simulink model "PruebaN9_sinRap"  (R2024b)
settings: Solver=ode45  StartTime=0.0  StopTime=10  RelTol=1e-3
values from neighbouring files (symbols this model uses):
  T = 10e-3    (= 0.01)    [Proceso.m]    (also in regdiagSISOsep.m = Reg.Ts; regdiagsep.m = Reg.Ts; regsep.m = Reg.Ts)
undefined symbols (not defined in the file or in its folder): N, RegDiag_Len2_ext, RegDiag_Len3_ext, RegDiag_Len4_ext, RegDiag_Len5_ext, RegDiag_Len6_ext, RegDiag_Len7_ext, RegDiag_Len8_ext, RegDiag_Len9_ext
libraries: cstblocks x12
settings Model: Creator=Guillem  LastModifiedBy=jroigro
settings SolverCC: AlgebraicLoopSolver=TrustRegion
settings DataIOCC: LimitDataPoints=on  SaveFormat=Array  SignalLoggingSaveFormat=ModelDataLogs  ReturnWorkspaceOutputs=off
settings OptimizationCC: BlockReduction=off  BooleanDataType=off  LifeSpan=inf
settings DebuggingCC: SaveWithParameterizedLinksMsg=none  UnderspecifiedInitializationDetection=Classic  MergeDetectMultiDrivingBlocksExec=none  SignalResolutionControl=TryResolveAllWithWarning  MultiTaskDSMMsg=warning  MultiTaskCondExecSysMsg=none  UnconnectedInputMsg=warning  UnconnectedOutputMsg=warning  UnconnectedLineMsg=warning  SFUnexpectedBacktrackingDiag=warning  SFNoUnconditionalDefaultTransitionDiag=warning  SFExecutionAtInitializationDiag=none  ArithmeticOperatorsInVariantConditions=warning
settings HardwareCC: ProdBitPerPointer=32  ProdBitPerSizeT=32  ProdBitPerPtrDiffT=32  ProdLargestAtomicFloat=None  ProdIntDivRoundTo=Undefined  ProdEndianess=Unspecified  ProdWordSize=32  ProdHWDeviceType=32-bit Generic  TargetUnknown=on
settings ModelReferenceCC: PropagateSignalLabelsOutOfModel=off
settings SFSimCC: SimUseLocalCustomCode=off  CustomCodeUndefinedFunction=UseInterfaceOnly
settings RTWCC: RTWUseLocalCustomCode=off  GPUComputeCapability=3.5
settings CodeAppCC: StateflowObjectComments=on
settings GRTTargetCC: TargetLangStandard=C89/C90 (ANSI)
settings ConfigComp: CovMetricSettings=dw  CovSaveCumulativeToWorkspaceVar=on  CovSaveSingleToWorkspaceVar=on  CovExternalEMLEnable=off

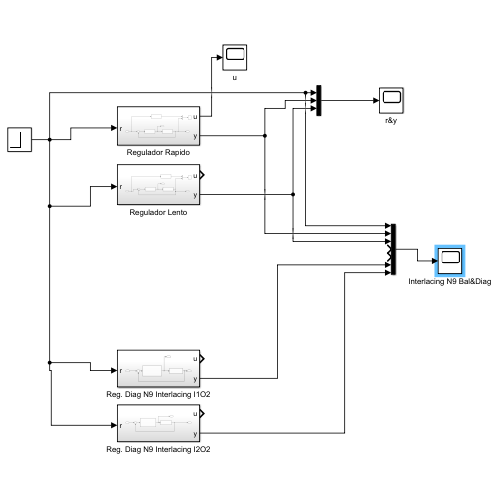
[thumbnail: Simulink's stored preview of the top-level diagram]
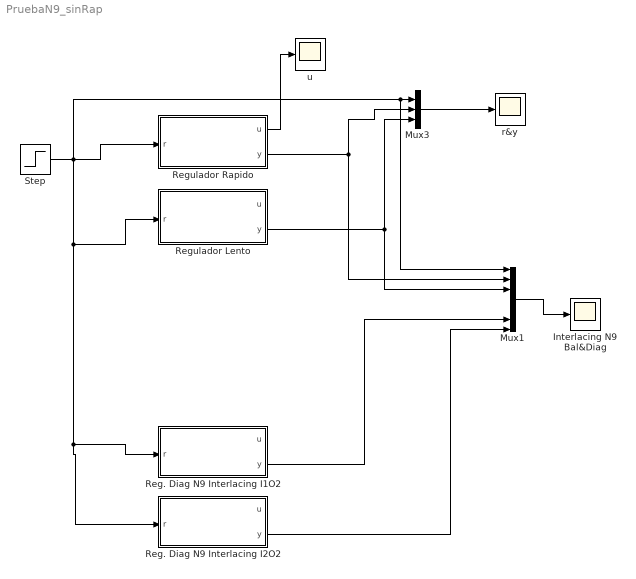
== system PruebaN9_sinRap ==
  Interlacing N9 Bal&Diag : Scope
  Mux1 : Mux  Inputs=7
  Mux3 : Mux  Inputs=3
  Reg. Diag N9 Interlacing I1O2 : Subsystem
  Reg. Diag N9 Interlacing I2O2 : Subsystem
  Regulador Lento : Subsystem
  Regulador Rapido : Subsystem
  Step : Step  Time=10  Before=1  After=2  SampleTime=0
  r&y : Scope
  u : Scope
  wires:
  Mux3/1 -> r&y/1
  Regulador Rapido/2(y) -> Mux1/2, Mux3/2
  Regulador Rapido/1(u) -> u/1
  Mux1/1 -> Interlacing N9 Bal&Diag/1
  Regulador Lento/2(y) -> Mux1/3, Mux3/3
  Step/1 -> Reg. Diag N9 Interlacing I1O2/1(r), Reg. Diag N9 Interlacing I2O2/1(r), Regulador Lento/1(r), Mux1/1, Mux3/1, Regulador Rapido/1(r)
  Reg. Diag N9 Interlacing I2O2/2(y) -> Mux1/7
  Reg. Diag N9 Interlacing I1O2/2(y) -> Mux1/6

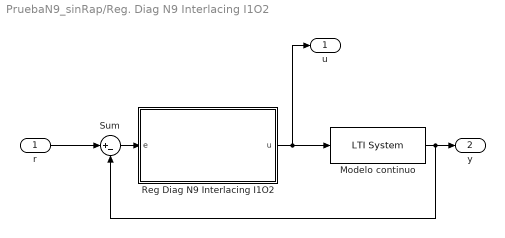
== system PruebaN9_sinRap/Reg. Diag N9 Interlacing I1O2 ==
  r : Inport
  Modelo continuo : cstblocks/LTI System  sys=Planta  IC=[]  PadeOrder=0
  Reg Diag N9 Interlacing I1O2 : Subsystem
  Sum : Sum  Inputs=|+-
  u : Outport
  y : Outport  Port=2
  wires:
  Reg Diag N9 Interlacing I1O2/1(u) -> Modelo continuo/1, u/1
  r/1 -> Sum/1
  Sum/1 -> Reg Diag N9 Interlacing I1O2/1(e)
  Modelo continuo/1 -> Sum/2, y/1

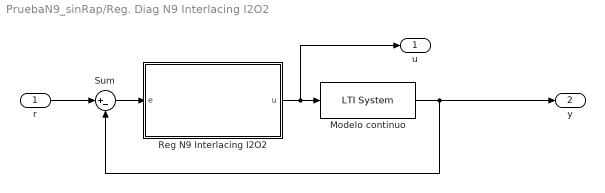
== system PruebaN9_sinRap/Reg. Diag N9 Interlacing I2O2 ==
  r : Inport
  Modelo continuo : cstblocks/LTI System  sys=Planta  IC=[]  PadeOrder=0
  Reg N9 Interlacing I2O2 : Subsystem
  Sum : Sum  Inputs=|+-
  u : Outport
  y : Outport  Port=2
  wires:
  Modelo continuo/1 -> Sum/2, y/1
  Reg N9 Interlacing I2O2/1(u) -> Modelo continuo/1, u/1
  r/1 -> Sum/1
  Sum/1 -> Reg N9 Interlacing I2O2/1(e)

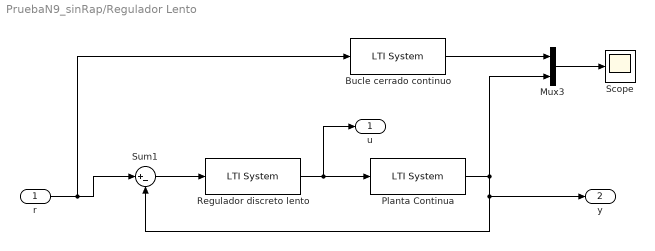
== system PruebaN9_sinRap/Regulador Lento ==
  r : Inport
  Bucle cerrado continuo : cstblocks/LTI System  sys=BC2  IC=[]  PadeOrder=0
  Mux3 : Mux  Inputs=2
  Planta Continua : cstblocks/LTI System  sys=Planta  IC=[]  PadeOrder=0
  Regulador discreto lento : cstblocks/LTI System  sys=GrN9  IC=[]  PadeOrder=0
  Scope : Scope
  Sum1 : Sum  Inputs=|+-
  u : Outport
  y : Outport  Port=2
  wires:
  r/1 -> Bucle cerrado continuo/1, Sum1/1
  Regulador discreto lento/1 -> u/1, Planta Continua/1
  Sum1/1 -> Regulador discreto lento/1
  Planta Continua/1 -> Sum1/2, y/1, Mux3/2
  Mux3/1 -> Scope/1
  Bucle cerrado continuo/1 -> Mux3/1

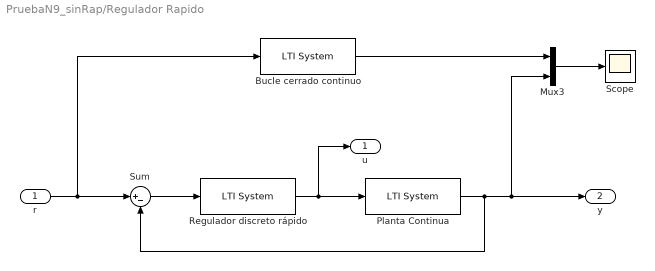
== system PruebaN9_sinRap/Regulador Rapido ==
  r : Inport
  Bucle cerrado continuo : cstblocks/LTI System  sys=BC1  IC=[]  PadeOrder=0
  Mux3 : Mux  Inputs=2
  Planta Continua : cstblocks/LTI System  sys=Planta  IC=[]  PadeOrder=0
  Regulador discreto rápido : cstblocks/LTI System  sys=Gr  IC=[]  PadeOrder=0
  Scope : Scope
  Sum : Sum  Inputs=|+-
  u : Outport
  y : Outport  Port=2
  wires:
  Regulador discreto rápido/1 -> u/1, Planta Continua/1
  Bucle cerrado continuo/1 -> Mux3/1
  Mux3/1 -> Scope/1
  Sum/1 -> Regulador discreto rápido/1
  Planta Continua/1 -> Mux3/2, y/1, Sum/2
  r/1 -> Sum/1, Bucle cerrado continuo/1

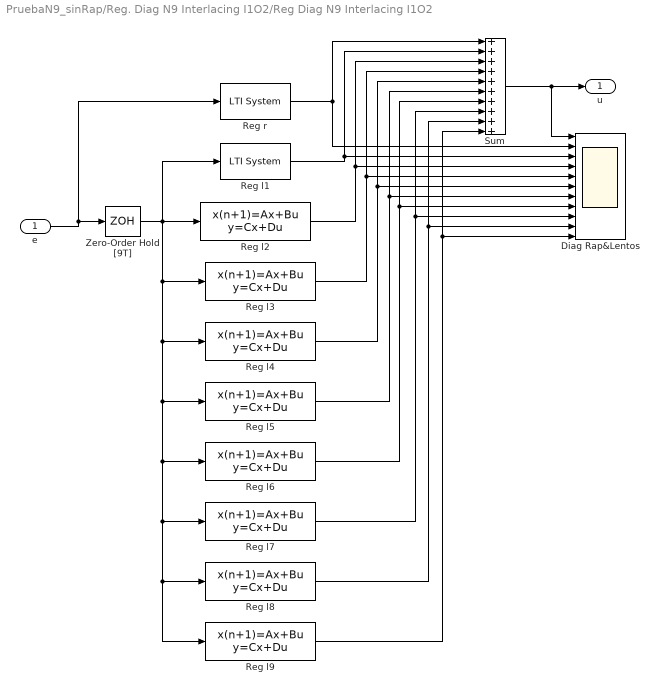
== system PruebaN9_sinRap/Reg. Diag N9 Interlacing I1O2/Reg Diag N9 Interlacing I1O2 ==
  e : Inport
  Diag Rap&Lentos : Scope  NumInputPorts=11
  Reg l1 : cstblocks/LTI System  sys=RegDiag_Len1_ext  IC=[]  PadeOrder=0
  Reg l2 : DiscreteStateSpace  A=RegDiag_Len2_ext.A  B=RegDiag_Len2_ext.B  C=RegDiag_Len2_ext.C  D=RegDiag_Len2_ext.D  SampleTime=[N*T,T]
  Reg l3 : DiscreteStateSpace  A=RegDiag_Len3_ext.A  B=RegDiag_Len3_ext.B  C=RegDiag_Len3_ext.C  D=RegDiag_Len3_ext.D  SampleTime=[N*T,2*T]
  Reg l4 : DiscreteStateSpace  A=RegDiag_Len4_ext.A  B=RegDiag_Len4_ext.B  C=RegDiag_Len4_ext.C  D=RegDiag_Len4_ext.D  SampleTime=[N*T,3*T]
  Reg l5 : DiscreteStateSpace  A=RegDiag_Len5_ext.A  B=RegDiag_Len5_ext.B  C=RegDiag_Len5_ext.C  D=RegDiag_Len5_ext.D  SampleTime=[N*T,4*T]
  Reg l6 : DiscreteStateSpace  A=RegDiag_Len6_ext.A  B=RegDiag_Len6_ext.B  C=RegDiag_Len6_ext.C  D=RegDiag_Len6_ext.D  SampleTime=[N*T,5*T]
  Reg l7 : DiscreteStateSpace  A=RegDiag_Len7_ext.A  B=RegDiag_Len7_ext.B  C=RegDiag_Len7_ext.C  D=RegDiag_Len7_ext.D  SampleTime=[N*T,6*T]
  Reg l8 : DiscreteStateSpace  A=RegDiag_Len8_ext.A  B=RegDiag_Len8_ext.B  C=RegDiag_Len8_ext.C  D=RegDiag_Len8_ext.D  SampleTime=[N*T,7*T]
  Reg l9 : DiscreteStateSpace  A=RegDiag_Len9_ext.A  B=RegDiag_Len9_ext.B  C=RegDiag_Len9_ext.C  D=RegDiag_Len9_ext.D  SampleTime=[N*T,8*T]
  Reg r : cstblocks/LTI System  sys=RegDiag_Rap  IC=[]  PadeOrder=0
  Sum : Sum  Inputs=++++++++++
  Zero-Order Hold [9T] : ZeroOrderHold  SampleTime=[N*T]
  u : Outport
  wires:
  Sum/1 -> u/1, Diag Rap&Lentos/1
  Reg l1/1 -> Sum/2, Diag Rap&Lentos/3
  Reg r/1 -> Diag Rap&Lentos/2, Sum/1
  e/1 -> Reg r/1, Zero-Order Hold [9T]/1
  Zero-Order Hold [9T]/1 -> Reg l9/1, Reg l8/1, Reg l7/1, Reg l6/1, Reg l5/1, Reg l4/1, Reg l3/1, Reg l1/1, Reg l2/1
  Reg l2/1 -> Sum/3, Diag Rap&Lentos/4
  Reg l3/1 -> Diag Rap&Lentos/5, Sum/4
  Reg l4/1 -> Sum/5, Diag Rap&Lentos/6
  Reg l5/1 -> Sum/6, Diag Rap&Lentos/7
  Reg l6/1 -> Sum/7, Diag Rap&Lentos/8
  Reg l7/1 -> Sum/8, Diag Rap&Lentos/9
  Reg l8/1 -> Diag Rap&Lentos/10, Sum/9
  Reg l9/1 -> Diag Rap&Lentos/11, Sum/10

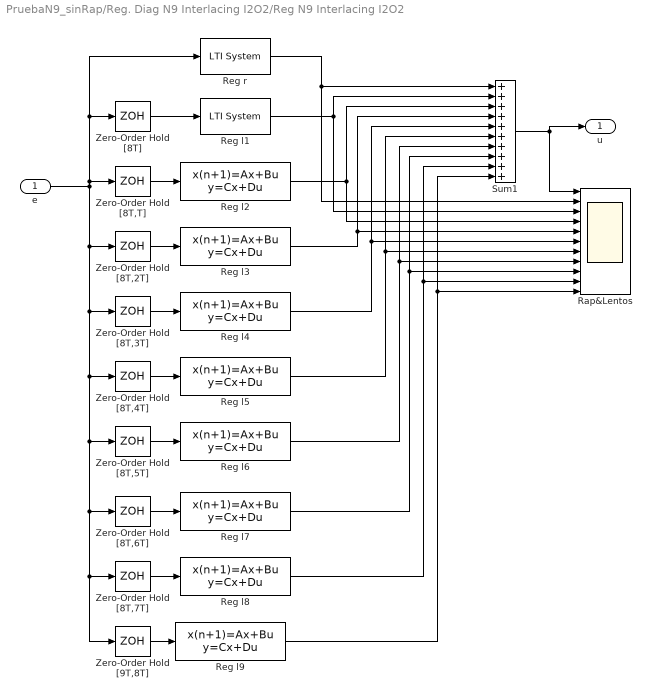
== system PruebaN9_sinRap/Reg. Diag N9 Interlacing I2O2/Reg N9 Interlacing I2O2 ==
  e : Inport
  Rap&Lentos : Scope  NumInputPorts=11
  Reg l1 : cstblocks/LTI System  sys=RegDiag_Len1_ext  IC=[]  PadeOrder=0
  Reg l2 : DiscreteStateSpace  A=RegDiag_Len2_ext.A  B=RegDiag_Len2_ext.B  C=RegDiag_Len2_ext.C  D=RegDiag_Len2_ext.D  SampleTime=[N*T,T]
  Reg l3 : DiscreteStateSpace  A=RegDiag_Len3_ext.A  B=RegDiag_Len3_ext.B  C=RegDiag_Len3_ext.C  D=RegDiag_Len3_ext.D  SampleTime=[N*T,2*T]
  Reg l4 : DiscreteStateSpace  A=RegDiag_Len4_ext.A  B=RegDiag_Len4_ext.B  C=RegDiag_Len4_ext.C  D=RegDiag_Len4_ext.D  SampleTime=[N*T,3*T]
  Reg l5 : DiscreteStateSpace  A=RegDiag_Len5_ext.A  B=RegDiag_Len5_ext.B  C=RegDiag_Len5_ext.C  D=RegDiag_Len5_ext.D  SampleTime=[N*T,4*T]
  Reg l6 : DiscreteStateSpace  A=RegDiag_Len6_ext.A  B=RegDiag_Len6_ext.B  C=RegDiag_Len6_ext.C  D=RegDiag_Len6_ext.D  SampleTime=[N*T,5*T]
  Reg l7 : DiscreteStateSpace  A=RegDiag_Len7_ext.A  B=RegDiag_Len7_ext.B  C=RegDiag_Len7_ext.C  D=RegDiag_Len7_ext.D  SampleTime=[N*T,6*T]
  Reg l8 : DiscreteStateSpace  A=RegDiag_Len8_ext.A  B=RegDiag_Len8_ext.B  C=RegDiag_Len8_ext.C  D=RegDiag_Len8_ext.D  SampleTime=[N*T,7*T]
  Reg l9 : DiscreteStateSpace  A=RegDiag_Len9_ext.A  B=RegDiag_Len9_ext.B  C=RegDiag_Len9_ext.C  D=RegDiag_Len9_ext.D  SampleTime=[N*T,8*T]
  Reg r : cstblocks/LTI System  sys=RegDiag_Rap  IC=[]  PadeOrder=0
  Sum1 : Sum  Inputs=++++++++++
  Zero-Order Hold [8T,2T] : ZeroOrderHold  SampleTime=[N*T,2*T]
  Zero-Order Hold [8T,3T] : ZeroOrderHold  SampleTime=[N*T,3*T]
  Zero-Order Hold [8T,4T] : ZeroOrderHold  SampleTime=[N*T,4*T]
  Zero-Order Hold [8T,5T] : ZeroOrderHold  SampleTime=[N*T,5*T]
  Zero-Order Hold [8T,6T] : ZeroOrderHold  SampleTime=[N*T,6*T]
  Zero-Order Hold [8T,7T] : ZeroOrderHold  SampleTime=[N*T,7*T]
  Zero-Order Hold [8T,T] : ZeroOrderHold  SampleTime=[N*T,T]
  Zero-Order Hold [8T] : ZeroOrderHold  SampleTime=[N*T]
  Zero-Order Hold [9T,8T] : ZeroOrderHold  SampleTime=[N*T,8*T]
  u : Outport
  wires:
  Reg l2/1 -> Rap&Lentos/4, Sum1/3
  Reg r/1 -> Rap&Lentos/2, Sum1/1
  Reg l1/1 -> Rap&Lentos/3, Sum1/2
  Sum1/1 -> u/1, Rap&Lentos/1
  Zero-Order Hold [8T,T]/1 -> Reg l2/1
  Zero-Order Hold [8T]/1 -> Reg l1/1
  Zero-Order Hold [8T,2T]/1 -> Reg l3/1
  Reg l3/1 -> Rap&Lentos/5, Sum1/4
  Zero-Order Hold [8T,3T]/1 -> Reg l4/1
  Reg l4/1 -> Sum1/5, Rap&Lentos/6
  Zero-Order Hold [8T,4T]/1 -> Reg l5/1
  Reg l5/1 -> Sum1/6, Rap&Lentos/7
  Zero-Order Hold [8T,5T]/1 -> Reg l6/1
  Reg l6/1 -> Sum1/7, Rap&Lentos/8
  Zero-Order Hold [8T,6T]/1 -> Reg l7/1
  e/1 -> Zero-Order Hold [8T,T]/1, Zero-Order Hold [8T]/1, Reg r/1, Zero-Order Hold [9T,8T]/1, Zero-Order Hold [8T,7T]/1, Zero-Order Hold [8T,6T]/1, Zero-Order Hold [8T,5T]/1, Zero-Order Hold [8T,4T]/1, Zero-Order Hold [8T,3T]/1, Zero-Order Hold [8T,2T]/1
  Reg l7/1 -> Sum1/8, Rap&Lentos/9
  Reg l8/1 -> Sum1/9, Rap&Lentos/10
  Zero-Order Hold [8T,7T]/1 -> Reg l8/1
  Zero-Order Hold [9T,8T]/1 -> Reg l9/1
  Reg l9/1 -> Rap&Lentos/11, Sum1/10
